simulink model "inverse_forward"  (R2021a)
settings: Solver=VariableStepAuto  StartTime=0.0  StopTime=10.0  RelTol=1e-3
undefined symbols (not defined in the file): Levenberg, Marquardt
libraries: robotcorelib x2, robotmaniplib x2
settings Model: Creator=ASUS  LastModifiedBy=ASUS

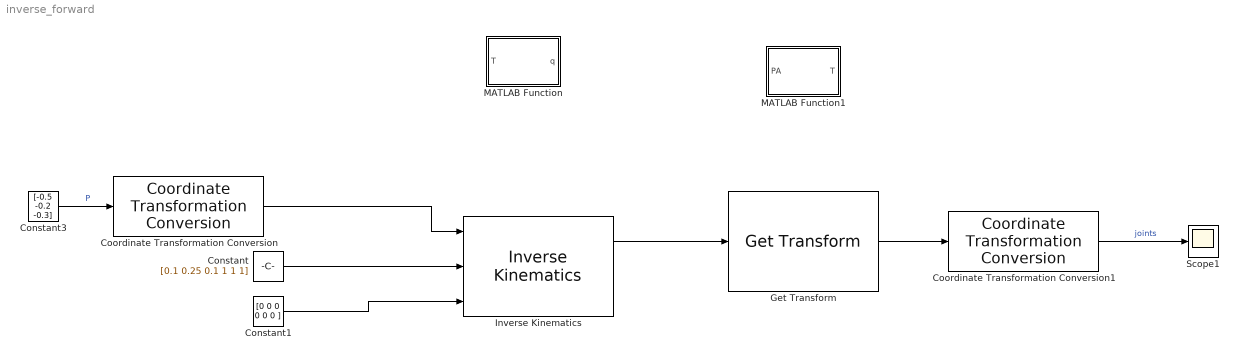
== system inverse_forward ==
  Constant : Constant  Value=[0.1 0.25 0.1 1 1 1]
  Constant1 : Constant  Value=[0 0 0 0 0 0 ]
  Constant3 : Constant  Value=[-0.5 -0.2 -0.3]
  Coordinate Transformation Conversion : robotcorelib/Coordinate Transformation Conversion  InputRepresentation=Translation Vector  InputEulerSequence=ZYX  ShowTrVecInputPort=on  OutputRepresentation=Homogeneous Transformation  OutputEulerSequence=ZYX  ShowTrVecOutputPort=on  SimulateUsing=Interpreted execution
      settings: SourceProductBaseCode=NV,RO,RR,UV
  Coordinate Transformation Conversion1 : robotcorelib/Coordinate Transformation Conversion  InputRepresentation=Homogeneous Transformation  InputEulerSequence=ZYX  ShowTrVecInputPort=on  OutputRepresentation=Translation Vector  OutputEulerSequence=ZYX  ShowTrVecOutputPort=on  SimulateUsing=Interpreted execution
      settings: SourceProductBaseCode=NV,RO,RR,UV
  Get Transform : robotmaniplib/Get Transform  RigidBodyTree=robot  SourceBody=tool0  TargetBody=world  SimulateUsing=Interpreted execution
  Inverse Kinematics : robotmaniplib/Inverse Kinematics  RigidBodyTree=robot  EndEffector=tool0  ShowInfo=on  SolverName=Levenberg-Marquardt  EnforceJointLimits=on  MaxIterations=1500  MaxTime=10  GradientTolerance=1e-3  SolutionTolerance=1e-3  StepTolerance=1e-14  ErrorChangeTolerance=1e-12  UseErrorDamping=on  DampingBias=0.0025  SimulateUsing=Interpreted execution
  MATLAB Function : MATLAB Function  TreatAsAtomicUnit=on
  MATLAB Function1 : MATLAB Function  TreatAsAtomicUnit=on
  Scope1 : Scope
  wires:
  Coordinate Transformation Conversion/1 -> Inverse Kinematics/1
  Get Transform/1 -> Coordinate Transformation Conversion1/1
  Constant1/1 -> Inverse Kinematics/3
  Inverse Kinematics/1 -> Get Transform/1
  Coordinate Transformation Conversion1/1 -> Scope1/1  "joints"
  Constant/1 -> Inverse Kinematics/2
  Constant3/1 -> Coordinate Transformation Conversion/1  "P"

== matlab function inverse_forward/MATLAB Function ==
  data: T input; q output
function q = fcn(T)

q = zeros(6,1);
q(1) = T(1,end);
q(2) = T(2,end);
q(3) = T(3,end);

R = T(1:3,1:3);
q(4:6) = rotm2eul(R)';

end

== matlab function inverse_forward/MATLAB Function1 ==
  data: PA input; T output
function T = fcn(PA)

T = se3(PA(4:6),"eul",PA(1:3));

end
